simulink model "TwoCharts"  (Simulink 7.4)
settings: Solver=ode45  StartTime=0.0  StopTime=10.0  RelTol=1e-3
settings Model: Creator=dread  LastModifiedBy=dread

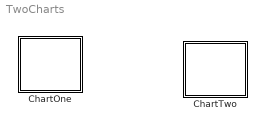
== system TwoCharts ==
  ChartOne : Stateflow chart
  ChartTwo : Stateflow chart

== stateflow chart ChartOne ==

== stateflow chart ChartTwo ==
